simulink model "Euler_w_mag"  (R2024b)
settings: Solver=FixedStepAuto  StartTime=0.0  StopTime=10  FixedStep=0.001  RelTol=1e-3
settings Model: Creator=cpero  LastModifiedBy=cpero

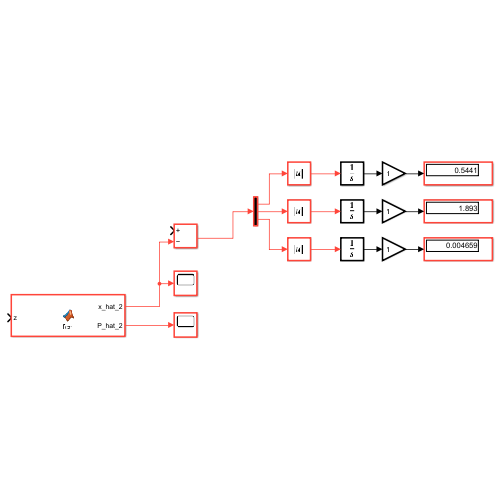
[thumbnail: Simulink's stored preview of the top-level diagram]
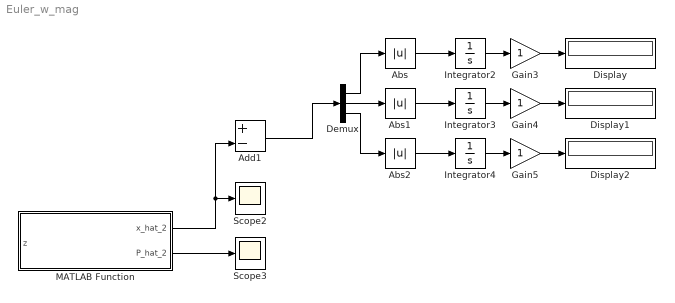
== system Euler_w_mag ==
  Abs : Abs  SaturateOnIntegerOverflow=off
  Abs1 : Abs  SaturateOnIntegerOverflow=off
  Abs2 : Abs  SaturateOnIntegerOverflow=off
  Add1 : Sum  Inputs=+-
  Demux : Demux  Outputs=3
  Display : Display
  Display1 : Display
  Display2 : Display
  Gain3 : Gain
  Gain4 : Gain
  Gain5 : Gain
  Integrator2 : Integrator
  Integrator3 : Integrator
  Integrator4 : Integrator
  MATLAB Function : MATLAB Function  TreatAsAtomicUnit=on
  Scope2 : Scope
  Scope3 : Scope
  wires:
  MATLAB Function/1(x_hat_2) -> Add1/2, Scope2/1
  MATLAB Function/2(P_hat_2) -> Scope3/1
  Add1/1 -> Demux/1
  Demux/1 -> Abs/1
  Integrator2/1 -> Gain3/1
  Gain3/1 -> Display/1
  Abs/1 -> Integrator2/1
  Demux/2 -> Abs1/1
  Integrator3/1 -> Gain4/1
  Abs1/1 -> Integrator3/1
  Gain4/1 -> Display1/1
  Abs2/1 -> Integrator4/1
  Integrator4/1 -> Gain5/1
  Demux/3 -> Abs2/1
  Gain5/1 -> Display2/1

== matlab function Euler_w_mag/MATLAB Function ==
  settings: updateMethod=DISCRETE
  data: z input; x_hat_2 output; P_hat_2 output
function [x_hat_2, P_hat_2] = fcn(z)

persistent x_hat_2_prior P_hat_2_prior

dt = 1e-3;

F = [1 dt 0.5*dt^2;
     0 1 dt
     0 0 1];
H = [1 0 0;
     0 0 1];

q = 0.01; % Process noise strength
Q = q * [dt^4/4, dt^3/2, dt^2/2; 
          dt^3/2, dt^2,   dt;    
          dt^2/2, dt,     1];
R = [1 0;
     0 10];

if isempty(x_hat_2_prior)
    x_hat_2_prior = [-1;2;0];
    P_hat_2_prior = 0.02*eye(3);
end

%Predict
x_hat_1 = F*x_hat_2_prior;
P_hat_1 = F*P_hat_2_prior*F' + Q;

%Update
y = z - H*x_hat_1;
S = H*P_hat_1*H' + R;
K = P_hat_1*H'*inv(S);
x_hat_2 = x_hat_1 + K*y;
P_hat_2 = (eye(3) - K*H)*P_hat_1;

x_hat_2_prior = x_hat_2;
P_hat_2_prior = P_hat_2;
